simulink model "substation"  (R2018a)
settings: Solver=ode15s  StartTime=0.0  StopTime=0.5  MaxStep=50e-6  RelTol=1e-3  EnableMultiTasking=on
undefined symbols (not defined in the file or in its folder): D1, Delta, Ts
libraries: powerlib x69, powerlib_extras x50
(part 2 of 2)

== system substation/Visualização5/wave-to-phasor ==
  fabc : Inport
  Demux1 : Demux  Outputs=3
  Mux : Mux  Inputs=3
  Mux1 : Mux  Inputs=3
  RMS : powerlib_extras/Measurements/Fourier  f1=60  n=1
  RMS1 : powerlib_extras/Measurements/Fourier  f1=60  n=1
  RMS2 : powerlib_extras/Measurements/Fourier  f1=60  n=1
  |Fabc| : Outport
  ang(Fabc) : Outport  Port=2
  wires:
  RMS/1 -> Mux/1  "|fa|"
  fabc/1 -> Demux1/1
  Demux1/1 -> RMS/1
  Demux1/2 -> RMS1/1
  Demux1/3 -> RMS2/1
  Mux/1 -> |Fabc|/1
  RMS1/1 -> Mux/2
  RMS2/1 -> Mux/3
  RMS2/2 -> Mux1/3
  RMS1/2 -> Mux1/2
  RMS/2 -> Mux1/1  "angIa"
  Mux1/1 -> ang(Fabc)/1

== system substation/Visualização5/wave-to-phasor1 ==
  fabc : Inport
  Demux1 : Demux  Outputs=3
  Mux : Mux  Inputs=3
  Mux1 : Mux  Inputs=3
  RMS : powerlib_extras/Measurements/Fourier  f1=60  n=1
  RMS1 : powerlib_extras/Measurements/Fourier  f1=60  n=1
  RMS2 : powerlib_extras/Measurements/Fourier  f1=60  n=1
  |Fabc| : Outport
  ang(Fabc) : Outport  Port=2
  wires:
  Mux1/1 -> ang(Fabc)/1
  RMS/2 -> Mux1/1  "angIa"
  RMS1/2 -> Mux1/2
  RMS2/2 -> Mux1/3
  RMS2/1 -> Mux/3
  RMS1/1 -> Mux/2
  Mux/1 -> |Fabc|/1
  Demux1/3 -> RMS2/1
  Demux1/2 -> RMS1/1
  Demux1/1 -> RMS/1
  fabc/1 -> Demux1/1
  RMS/1 -> Mux/1  "|fa|"

== system substation/Visualização6/wave-to-phasor ==
  fabc : Inport
  Demux1 : Demux  Outputs=3
  Mux : Mux  Inputs=3
  Mux1 : Mux  Inputs=3
  RMS : powerlib_extras/Measurements/Fourier  f1=60  n=1
  RMS1 : powerlib_extras/Measurements/Fourier  f1=60  n=1
  RMS2 : powerlib_extras/Measurements/Fourier  f1=60  n=1
  |Fabc| : Outport
  ang(Fabc) : Outport  Port=2
  wires:
  RMS/1 -> Mux/1  "|fa|"
  fabc/1 -> Demux1/1
  Demux1/1 -> RMS/1
  Demux1/2 -> RMS1/1
  Demux1/3 -> RMS2/1
  Mux/1 -> |Fabc|/1
  RMS1/1 -> Mux/2
  RMS2/1 -> Mux/3
  RMS2/2 -> Mux1/3
  RMS1/2 -> Mux1/2
  RMS/2 -> Mux1/1  "angIa"
  Mux1/1 -> ang(Fabc)/1

== system substation/Visualização6/wave-to-phasor1 ==
  fabc : Inport
  Demux1 : Demux  Outputs=3
  Mux : Mux  Inputs=3
  Mux1 : Mux  Inputs=3
  RMS : powerlib_extras/Measurements/Fourier  f1=60  n=1
  RMS1 : powerlib_extras/Measurements/Fourier  f1=60  n=1
  RMS2 : powerlib_extras/Measurements/Fourier  f1=60  n=1
  |Fabc| : Outport
  ang(Fabc) : Outport  Port=2
  wires:
  Mux1/1 -> ang(Fabc)/1
  RMS/2 -> Mux1/1  "angIa"
  RMS1/2 -> Mux1/2
  RMS2/2 -> Mux1/3
  RMS2/1 -> Mux/3
  RMS1/1 -> Mux/2
  Mux/1 -> |Fabc|/1
  Demux1/3 -> RMS2/1
  Demux1/2 -> RMS1/1
  Demux1/1 -> RMS/1
  fabc/1 -> Demux1/1
  RMS/1 -> Mux/1  "|fa|"

== system substation/protecao 1/wave-to-phasor ==
  fabc : Inport
  Demux1 : Demux  Outputs=3
  Mux : Mux  Inputs=3
  Mux1 : Mux  Inputs=3
  RMS : powerlib_extras/Measurements/Fourier  f1=60  n=1
  RMS1 : powerlib_extras/Measurements/Fourier  f1=60  n=1
  RMS2 : powerlib_extras/Measurements/Fourier  f1=60  n=1
  |Fabc| : Outport
  ang(Fabc) : Outport  Port=2
  wires:
  Mux1/1 -> ang(Fabc)/1
  RMS/2 -> Mux1/1  "angIa"
  RMS1/2 -> Mux1/2
  RMS2/2 -> Mux1/3
  RMS2/1 -> Mux/3
  RMS1/1 -> Mux/2
  Mux/1 -> |Fabc|/1
  Demux1/3 -> RMS2/1
  Demux1/2 -> RMS1/1
  Demux1/1 -> RMS/1
  fabc/1 -> Demux1/1
  RMS/1 -> Mux/1  "|fa|"

== system substation/protecao 50/wave-to-phasor ==
  fabc : Inport
  Demux1 : Demux  Outputs=3
  Mux : Mux  Inputs=3
  Mux1 : Mux  Inputs=3
  RMS : powerlib_extras/Measurements/Fourier  f1=60  n=1
  RMS1 : powerlib_extras/Measurements/Fourier  f1=60  n=1
  RMS2 : powerlib_extras/Measurements/Fourier  f1=60  n=1
  |Fabc| : Outport
  ang(Fabc) : Outport  Port=2
  wires:
  RMS/1 -> Mux/1  "|fa|"
  fabc/1 -> Demux1/1
  Demux1/1 -> RMS/1
  Demux1/2 -> RMS1/1
  Demux1/3 -> RMS2/1
  Mux/1 -> |Fabc|/1
  RMS1/1 -> Mux/2
  RMS2/1 -> Mux/3
  RMS2/2 -> Mux1/3
  RMS1/2 -> Mux1/2
  RMS/2 -> Mux1/1  "angIa"
  Mux1/1 -> ang(Fabc)/1

== matlab function substation/Operation ==
  data: s_7M1 output; s_7M2 output; s_7M4 output; s_7M5 output; s_7M6 output; t input; t0 output
function [s_7M1, s_7M2, s_7M4, s_7M5, s_7M6, t0] = fcn(t)
persistent flag s_7M1_p s_7M2_p s_7M4_p s_7M5_p s_7M6_p t0_p;

if isempty(flag)
    % Inicializa variáveis persistentes
    s_7M1_p = 1;
    s_7M2_p = 1;
    s_7M4_p = 1;
    s_7M5_p = 1;
    s_7M6_p = 0;
    t0_p = 0;
    flag = 1; % Marca que foi inicializado
end

% Atualiza variáveis quando t >= 0
if ( (t >= 0) && (t < 0.1))
    s_7M1_p = 1;
    s_7M2_p = 1;
    s_7M4_p = 1;
    s_7M5_p = 1;
    s_7M6_p = 0;
    t0_p = t;
else
    s_7M1_p = 0;
    s_7M2_p = 1;
    s_7M4_p = 1;
    s_7M5_p = 1;
    s_7M6_p = 0;
    t0_p = t;
end

% Retorna os valores atualizados
s_7M1 = s_7M1_p;
s_7M2 = s_7M2_p;
s_7M4 = s_7M4_p;
s_7M5 = s_7M5_p;
s_7M6 = s_7M6_p;
t0 = t0_p;
end
% function [s_7M1,s_7M2,s_7M4,s_7M5,s_7M6, t0] = fcn(t)
% persistent flag;
% if isempty(flag)
%     s_7M1 = 0;
%     s_7M2 = 1;
%     s_7M4 = 1;
%     s_7M5 = 1;
%     s_7M6 = 0;
%     t0 = 0;
% 
%     flag = 0;
% end
% if ( t >= 0 )
%     s_7M1 = 0;
%     s_7M2 = 1;
%     s_7M4 = 1;
%     s_7M5 = 1;
%     s_7M6 = 0;
%     t0 = t;
% end
% end
